simulink library "seg_display"  (R2023b)
settings: Solver=VariableStepAuto  StartTime=0.0  StopTime=10.0  RelTol=1e-3
settings Model: Creator=mueller.chris-it22  LastModifiedBy=kilia

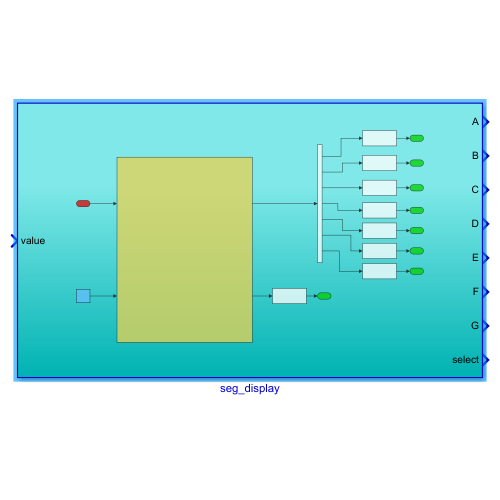
[thumbnail: Simulink's stored preview of the top-level diagram]
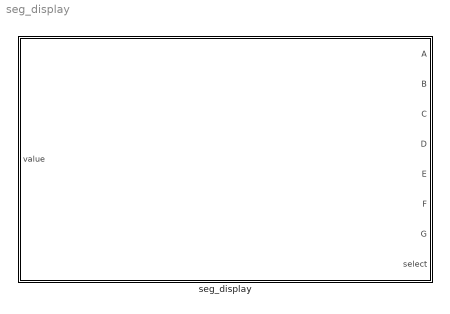
== system seg_display ==
  seg_display : Subsystem

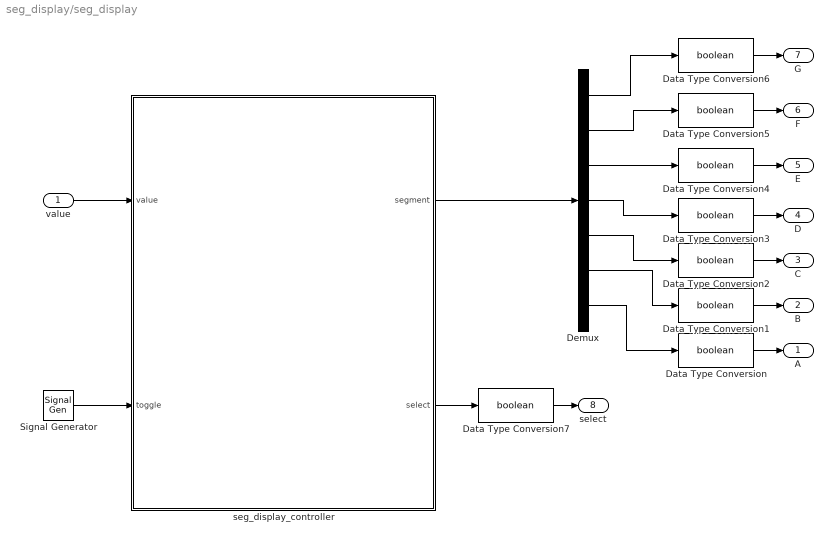
== system seg_display/seg_display ==
  value : Inport
  Data Type Conversion{,1..7} (8 alike) : DataTypeConversion  OutDataTypeStr=boolean  SaturateOnIntegerOverflow=off  RndMeth=Floor
  Demux : Demux  Outputs=7
  Signal Generator : SignalGenerator  WaveForm=square  Frequency=15
  seg_display_controller : MATLAB Function  TreatAsAtomicUnit=on
  A : Outport
  B : Outport  Port=2
  C : Outport  Port=3
  D : Outport  Port=4
  E : Outport  Port=5
  F : Outport  Port=6
  G : Outport  Port=7
  select : Outport  Port=8
  wires:
  seg_display_controller/1(segment) -> Demux/1
  seg_display_controller/2(select) -> Data Type Conversion7/1
  value/1 -> seg_display_controller/1(value)
  Demux/1 -> Data Type Conversion6/1
  Demux/2 -> Data Type Conversion5/1
  Demux/3 -> Data Type Conversion4/1
  Demux/4 -> Data Type Conversion3/1
  Demux/5 -> Data Type Conversion2/1
  Demux/6 -> Data Type Conversion1/1
  Demux/7 -> Data Type Conversion/1
  Data Type Conversion7/1 -> select/1
  Signal Generator/1 -> seg_display_controller/2(toggle)
  Data Type Conversion6/1 -> G/1
  Data Type Conversion5/1 -> F/1
  Data Type Conversion4/1 -> E/1
  Data Type Conversion3/1 -> D/1
  Data Type Conversion2/1 -> C/1
  Data Type Conversion1/1 -> B/1
  Data Type Conversion/1 -> A/1

== matlab function seg_display/seg_display_controller ==
  data: segment output; value input; toggle input; select output
function [segment, select] = SevenSegmentControl(value, toggle)
% Eingänge:
% value: Zahlenwert (0–99), der angezeigt werden soll
% toggle: Umschaltsignal (0 oder 1) zum Wechsel zwischen Zehner- und Einerstelle

% Ausgänge:
% segment: 8-Bit-Signal für die Segmente (a-g und dp)
% select: 2-Bit-Signal zur Aktivierung eines Displays

% Begrenzung des Werts auf den Bereich 0–99
value = max(0, min(99, value));

% Segment-Codes für 0–9 (a-g, dp: [abcdefg.dp])
segments_tens = [
    1,0,0,0,0,0,0; % 0
    1,1,1,1,0,0,1; % 1
    0,1,0,0,1,0,0; % 2
    1,1,1,0,0,0,0; % 3
    0,0,1,1,0,0,1; % 4
    0,0,1,0,0,1,0; % 5
    0,0,0,0,0,1,0; % 6
    1,1,1,1,0,0,0; % 7
    0,0,0,0,0,0,0; % 8
    0,0,1,0,0,0,0; % 9
];

segments_ones = [
    0,1,1,1,1,1,1; % 0
    0,0,0,0,1,1,0; % 1
    1,0,1,1,0,1,1; % 2
    0,0,0,1,1,1,1; % 3
    1,1,0,0,1,1,0; % 4
    1,1,0,1,1,0,1; % 5
    1,1,1,1,1,0,1; % 6
    0,0,0,0,1,1,1; % 7
    1,1,1,1,1,1,1; % 8
    1,1,0,1,1,1,1; % 9
];

% Zerlege den Wert in Zehner- und Einerstelle
tens = floor(value / 10);
ones = mod(value, 10);

% Anzeigelogik basierend auf toggle
if toggle == 1
    segment = reshape(segments_tens(tens + 1,:), [7, 1]); % Zehnerstelle
    select = 1; % Aktiviert das erste Display
else
    segment = reshape(segments_ones(ones + 1,:), [7, 1]); % Einerstelle
    select = 0; % Aktiviert das zweite Display
end
end
